simulink model "Closedloop2"  (R2015b)
settings: Solver=VariableStepAuto  StartTime=0.0  StopTime=600  RelTol=1e-3
values from neighbouring files (symbols this model uses):
  A = [a11 a12 a13;a21 a22 a23;a31 a32 a33]    [ControllerWT1.m]    (also in ControllerWT2.m; Robustness.m)
  a11 = -Cr/Jr    [ControllerWT1.m]    (also in ControllerWT2.m; Robustness.m; Run_me.m = -0.000211148648649)
  a12 = 0    [ControllerWT1.m]    (also in ControllerWT2.m; Robustness.m; Run_me.m)
  a13 = -1/Jr    [ControllerWT1.m]    (also in ControllerWT2.m; Robustness.m; Run_me.m = -3.37837837838e-07)
  a21 = 0    [ControllerWT1.m]    (also in ControllerWT2.m; Robustness.m; Run_me.m)
  a22 = -Cg/Jg    (= -0.000942755863941)    [ControllerWT1.m]    (also in ControllerWT2.m = -Cg/Jg; Robustness.m = -Cg/Jg; Run_me.m)
  a23 = 1/ng/Jg    (= 0.000214347948375)    [ControllerWT1.m]    (also in ControllerWT2.m = 1/ng/Jg; Robustness.m = 1/ng/Jg; Run_me.m)
  a31 = Kls-Cls*Cr/Jr    [ControllerWT1.m]    (also in ControllerWT2.m; Robustness.m; Run_me.m = 559978.885135)
  a32 = (Cls*Cg/Jg-Kls)/ng    [ControllerWT1.m]    (also in ControllerWT2.m; Robustness.m; Run_me.m = -6365.09662267)
  a33 = -Cls*(Jr+ng^2*Jg)/(ng^2*Jg*Jr)    [ControllerWT1.m]    (also in ControllerWT2.m; Robustness.m; Run_me.m = -0.277457913694)
  B = [b11*10^6 b12*10^4;b21*10^6 b22*10^4;b31*10^6 b32*10^4]    [ControllerWT1.m]    (also in ControllerWT2.m; Robustness.m = [0 b11*10^6 b12*10^4;0 b21*10^6 b22*10^4;0 b31*10^6 b32*10^4)
  b11 = 1/Jr    [ControllerWT1.m]    (also in ControllerWT2.m; Robustness.m; Run_me.m = 3.37837837838e-07)
  b12 = 0    [ControllerWT1.m]    (also in ControllerWT2.m; Robustness.m; Run_me.m)
  b21 = 0    [ControllerWT1.m]    (also in ControllerWT2.m; Robustness.m; Run_me.m)
  b22 = -1/Jg    (= -0.0188551172788)    [ControllerWT1.m]    (also in ControllerWT2.m = -1/Jg; Robustness.m = -1/Jg; Run_me.m)
  b31 = Cls/Jr    [ControllerWT1.m]    (also in ControllerWT2.m; Robustness.m; Run_me.m = 0.0337837837838)
  b32 = Cls/ng/Jg    [ControllerWT1.m]    (also in ControllerWT2.m; Robustness.m; Run_me.m = 21.4347948375)
  C = [0 0 0;1 0 0;a21 a22 a23;0 0 0;0 1 0]    [ControllerWT1.m]    (also in ControllerWT2.m; Robustness.m = [0 0 0;1 0 0;a21 a22 a23;1 0 0;0 0 0;0 1 0])
  Cp = xlsread(filename)    [Run_me.m]
  D = [0 1;0 0;b21*10^6 b22*10^4;1 0;0 0]    [ControllerWT1.m]    (also in ControllerWT2.m; Robustness.m = [0 0 1;0 0 0;0 b21*10^6 b22*10^4;-lambda_opt/R 0 0;0 1 0;0 0)
  lambda_opt = 7.1    [ControllerWT1.m]    (also in ControllerWT2.m; Robustness.m; Run_me.m)
  R = ureal('Rho',35,'Percentage',1)    [ControllerWT1.m]    (also in ControllerWT2.m; Robustness.m = ureal('Rho',35,'Percentage',15); Run_me.m = 35)
  Rho = ureal('Rho',1.225,'Percentage',1)    [ControllerWT1.m]    (also in ControllerWT2.m; Robustness.m = ureal('Rho',1.225,'Percentage',15); Run_me.m = 1.225)
  vf = xlsread(filename)    [Run_me.m]
settings Model: Creator=alino  LastModifiedBy=alino

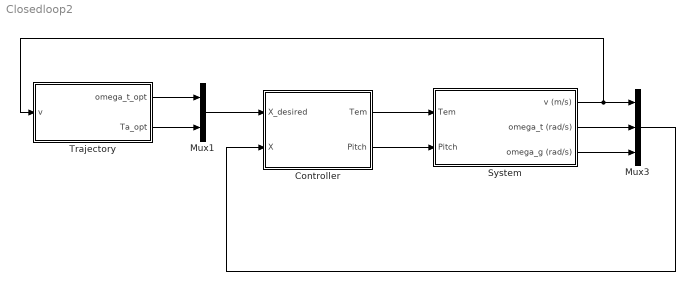
== system Closedloop2 ==
  Controller : Subsystem
  Mux1 : Mux  Inputs=2
  Mux3 : Mux  Inputs=3
  System : Subsystem
  Trajectory : Subsystem
  wires:
  Mux3/1 -> Controller/2(X)
  Mux1/1 -> Controller/1(X_desired)
  Trajectory/1(omega_t_opt) -> Mux1/1
  Controller/1(Tem) -> System/1(Tem)
  Controller/2(Pitch) -> System/2(Pitch)
  System/3(omega_g (rad/s)) -> Mux3/3
  System/2(omega_t (rad/s)) -> Mux3/2
  System/1(v (m/s)) -> Trajectory/1(v), Mux3/1
  Trajectory/2(Ta_opt) -> Mux1/2

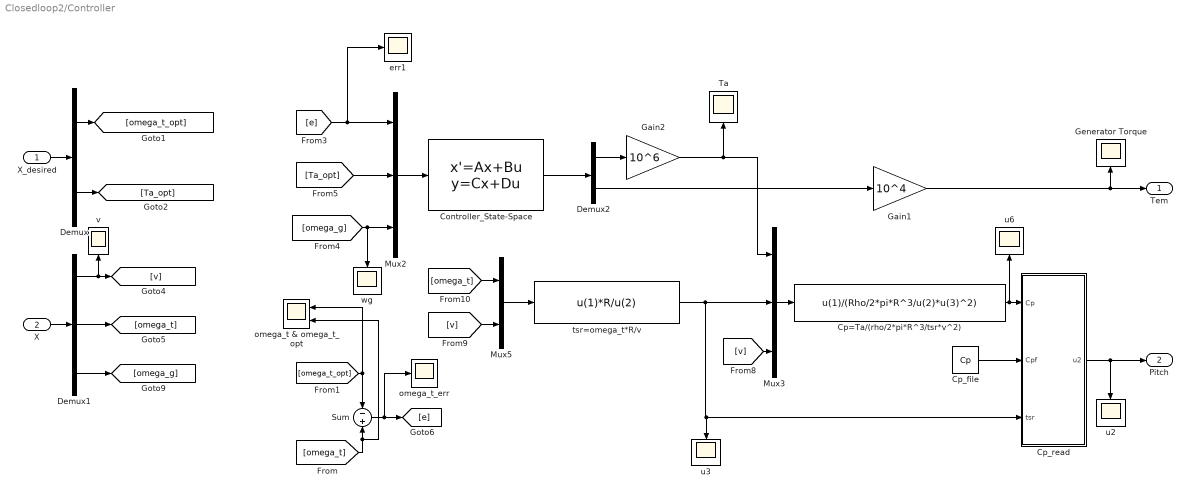
== system Closedloop2/Controller ==
  X_desired : Inport
  X : Inport  Port=2
  Controller_State-Space : StateSpace  A=A  B=B  C=C  D=D  X0=0
  Cp=Ta/(rho/2*pi*R^3/tsr*v^2) : Fcn  Expr=u(1)/(Rho/2*pi*R^3/u(2)*u(3)^2)
  Cp_file : Constant  Value=Cp
  Cp_read : MATLAB Function  TreatAsAtomicUnit=on
  Demux : Demux  Outputs=2
  Demux1 : Demux  Outputs=3
  Demux2 : Demux  Outputs=2
  Gain1 : Gain  Gain=10^4
  Gain2 : Gain  Gain=10^6
  Generator Torque : Scope
  Mux2 : Mux  Inputs=3
  Mux3 : Mux  Inputs=3
  Mux5 : Mux  Inputs=2
  Sum : Sum  Inputs=-+
  Ta : Scope
  err1 : Scope
  omega_t & omega_t_opt : Scope  NumInputPorts=2
  omega_t_err : Scope
  tsr=omega_t*R/v : Fcn  Expr=u(1)*R/u(2)
  u2 : Scope
  u3 : Scope
  u6 : Scope
  v : Scope
  wg : Scope
  Tem : Outport
  Pitch : Outport  Port=2
  wires:
  X_desired/1 -> Demux/1
  X/1 -> Demux1/1
  Demux/1 -> [omega_t_opt]
  Demux/2 -> [Ta_opt]
  Demux1/1 -> v/1, [v]
  Demux1/2 -> [omega_t]
  Demux1/3 -> [omega_g]
  Cp_read/1(u2) -> Pitch/1, u2/1
  Sum/1 -> omega_t_err/1, [e]
  [omega_t] -> omega_t & omega_t_opt/2, Sum/2
  [omega_t_opt] -> omega_t & omega_t_opt/1, Sum/1
  [v] -> Mux3/3
  Mux5/1 -> tsr=omega_t*R/v/1
  [v] -> Mux5/2
  [omega_t] -> Mux5/1
  tsr=omega_t*R/v/1 -> Cp_read/3(tsr), u3/1, Mux3/2
  Demux2/2 -> Gain1/1
  [Ta_opt] -> Mux2/2
  Gain2/1 -> Mux3/1, Ta/1
  Mux3/1 -> Cp=Ta/(rho/2*pi*R^3/tsr*v^2)/1
  Cp=Ta/(rho/2*pi*R^3/tsr*v^2)/1 -> u6/1, Cp_read/1(Cp)
  Cp_file/1 -> Cp_read/2(Cpf)
  Gain1/1 -> Generator Torque/1, Tem/1
  [omega_g] -> Mux2/3, wg/1
  Demux2/1 -> Gain2/1
  Controller_State-Space/1 -> Demux2/1
  Mux2/1 -> Controller_State-Space/1
  [e] -> Mux2/1, err1/1

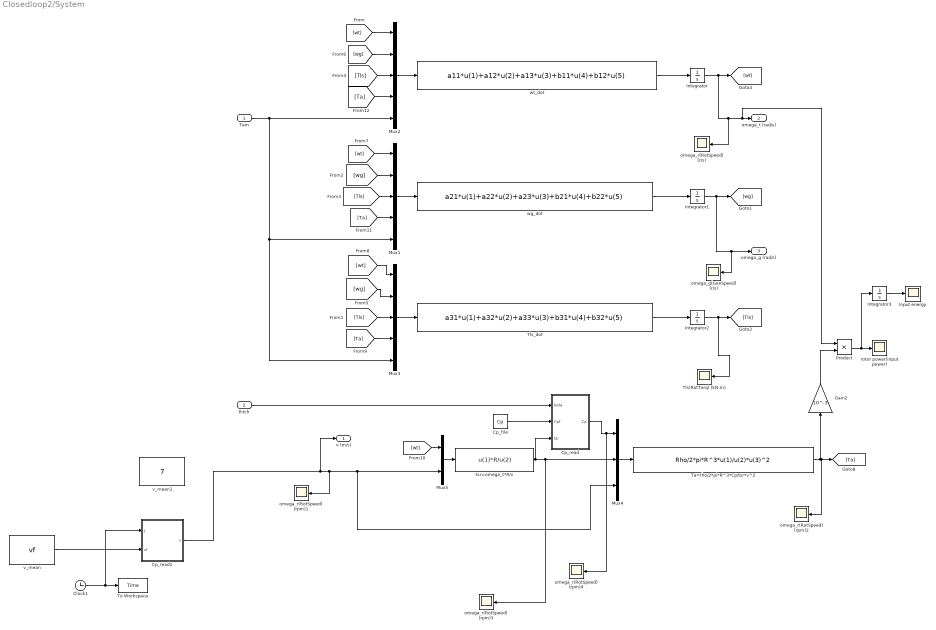
== system Closedloop2/System ==
  Tem : Inport
  Pitch : Inport  Port=2
  Clock1 : Clock
  Cp_file : Constant  Value=Cp
  Cp_read : MATLAB Function  TreatAsAtomicUnit=on
  Cp_read1 : MATLAB Function  TreatAsAtomicUnit=on
  Gain2 : Gain  Gain=10^-3
  Input energy : Scope
  Integrator : Integrator  InitialCondition=2
  Integrator1 : Integrator  InitialCondition=2
  Integrator2 : Integrator
  Integrator3 : Integrator
  Mux1 : Mux  Inputs=5
  Mux2 : Mux  Inputs=5
  Mux3 : Mux  Inputs=5
  Mux4 : Mux  Inputs=3
  Mux5 : Mux  Inputs=2
  Product : Product
  Ta=rho/2*pi*R^3*Cp/tsr*v^2 : Fcn  Expr=Rho/2*pi*R^3*u(1)/u(2)*u(3)^2
  Tls(RotTorq) (kN.m) : Scope
  Tls_dot : Fcn  Expr=a31*u(1)+a32*u(2)+a33*u(3)+b31*u(4)+b32*u(5)
  To Workspace : ToWorkspace  VariableName=Time  SampleTime=-1
  omega_g(GenSpeed) (r/s) : Scope
  omega_r(RotSpeed) (r/s) : Scope
  omega_r(RotSpeed) (rpm){1..4} (4 alike) : Scope
  rotor power(input power) : Scope
  tsr=omega_t*R/v : Fcn  Expr=u(1)*R/u(2)
  v_mean : Constant  Value=vf
  v_mean1 : Constant  Value=7
  wg_dot : Fcn  Expr=a21*u(1)+a22*u(2)+a23*u(3)+b21*u(4)+b22*u(5)
  wt_dot : Fcn  Expr=a11*u(1)+a12*u(2)+a13*u(3)+b11*u(4)+b12*u(5)
  v (m/s) : Outport
  omega_t (rad/s) : Outport  Port=2
  omega_g (rad/s) : Outport  Port=3
  wires:
  Integrator/1 -> Product/1, omega_t (rad/s)/1, omega_r(RotSpeed) (r/s)/1, [wt]
  Integrator1/1 -> omega_g(GenSpeed) (r/s)/1, omega_g (rad/s)/1, [wg]
  Integrator2/1 -> Tls(RotTorq) (kN.m)/1, [Tls]
  Pitch/1 -> Cp_read/1(beta)
  Mux2/1 -> wt_dot/1
  Mux1/1 -> wg_dot/1
  Mux3/1 -> Tls_dot/1
  wt_dot/1 -> Integrator/1
  [wt] -> Mux2/1
  wg_dot/1 -> Integrator1/1
  Tls_dot/1 -> Integrator2/1
  [wt] -> Mux3/1
  [wg] -> Mux1/2
  [Tls] -> Mux3/3
  [Tls] -> Mux1/3
  [Tls] -> Mux2/3
  [wg] -> Mux3/2
  [wg] -> Mux2/2
  [wt] -> Mux1/1
  Tem/1 -> Mux3/5, Mux1/5, Mux2/5
  Mux4/1 -> Ta=rho/2*pi*R^3*Cp/tsr*v^2/1
  Cp_read1/1(v) -> v (m/s)/1, omega_r(RotSpeed) (rpm)1/1, Mux4/3, Mux5/2
  Mux5/1 -> tsr=omega_t*R/v/1
  [wt] -> Mux5/1
  tsr=omega_t*R/v/1 -> omega_r(RotSpeed) (rpm)3/1, Mux4/2, Cp_read/3(tsr)
  Ta=rho/2*pi*R^3*Cp/tsr*v^2/1 -> [Ta], omega_r(RotSpeed) (rpm)2/1, Gain2/1
  Cp_read/1(Cp) -> omega_r(RotSpeed) (rpm)4/1, Mux4/1
  Cp_file/1 -> Cp_read/2(Cpf)
  [Ta] -> Mux3/4
  [Ta] -> Mux1/4
  [Ta] -> Mux2/4
  Clock1/1 -> Cp_read1/1(t), To Workspace/1
  v_mean/1 -> Cp_read1/2(vf)
  Product/1 -> Integrator3/1, rotor power(input power)/1
  Gain2/1 -> Product/2
  Integrator3/1 -> Input energy/1

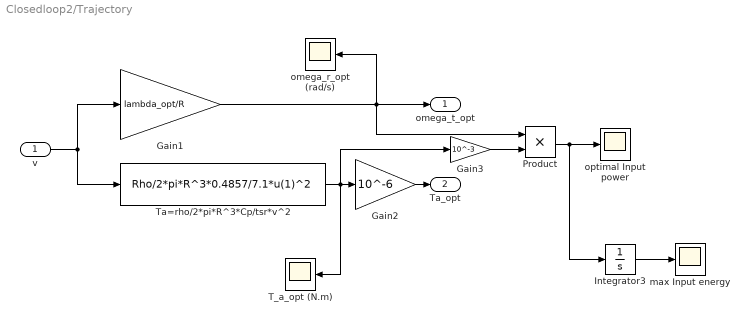
== system Closedloop2/Trajectory ==
  v : Inport
  Gain1 : Gain  Gain=lambda_opt/R
  Gain2 : Gain  Gain=10^-6
  Gain3 : Gain  Gain=10^-3
  Integrator3 : Integrator
  Product : Product
  T_a_opt (N.m) : Scope
  Ta=rho/2*pi*R^3*Cp/tsr*v^2 : Fcn  Expr=Rho/2*pi*R^3*0.4857/7.1*u(1)^2
  max Input energy : Scope
  omega_r_opt (rad/s) : Scope
  optimal Input power : Scope
  omega_t_opt : Outport
  Ta_opt : Outport  Port=2
  wires:
  v/1 -> Gain1/1, Ta=rho/2*pi*R^3*Cp/tsr*v^2/1
  Gain1/1 -> Product/1, omega_r_opt (rad/s)/1, omega_t_opt/1
  Ta=rho/2*pi*R^3*Cp/tsr*v^2/1 -> Gain3/1, T_a_opt (N.m)/1, Gain2/1
  Gain2/1 -> Ta_opt/1
  Gain3/1 -> Product/2
  Product/1 -> Integrator3/1, optimal Input power/1
  Integrator3/1 -> max Input energy/1

== matlab function Closedloop2/Controller/Cp_read ==
  data: Cp input; u2 output; Cpf input; tsr input
function u2 = fcn(Cp,Cpf,tsr)
    tsr=floor(tsr*10+0.5);
    beta=2;
    if (Cp>0) && (Cp<0.4857) && (tsr<20) && (tsr>0)
        i=90;
        while (Cp>Cpf(i,tsr))
            i=i-1;
            if i==0 
                break; 
            end
        end
        if i~=0
            p=(Cp-Cpf(i+1,tsr))/(Cpf(i,tsr)-Cpf(i+1,tsr));
            beta=(i-p);
        end
    end
    u2=beta;
end

== matlab function Closedloop2/System/Cp_read1 ==
  data: t input; v output; vf input
function v = fcn(t,vf)
    v=vf(floor(0.5*t)+1);
end

== matlab function Closedloop2/System/Cp_read ==
  data: beta input; Cpf input; Cp output; tsr input
function Cp = fcn(beta,Cpf,tsr)

    Cp=0;
    if (beta>=0) && (beta<90) && (tsr<20) && (tsr>0.1)
        beta1=floor(beta)+1;
        tsr1=floor(tsr*10);
        beta2=beta1+1;
        tsr2=tsr1+1;
        betap=beta-floor(beta);
        tsrp=tsr*10-floor(tsr*10);
        Cp1=Cpf(beta1,tsr1)+betap*(Cpf(beta2,tsr1)-Cpf(beta1,tsr1));
        Cp2=Cpf(beta1,tsr2)+betap*(Cpf(beta2,tsr2)-Cpf(beta1,tsr2));
        Cp=tsrp*(Cp2-Cp1)+Cp1;
    end
end
